simulink model "MotorPlant_23_lab2_discrete"  (R2019b)
settings: Solver=FixedStepAuto  StartTime=0.0  StopTime=2  FixedStep=0.001  RelTol=1e-3
settings Model: Creator=cmcaradi  LastModifiedBy=Laura

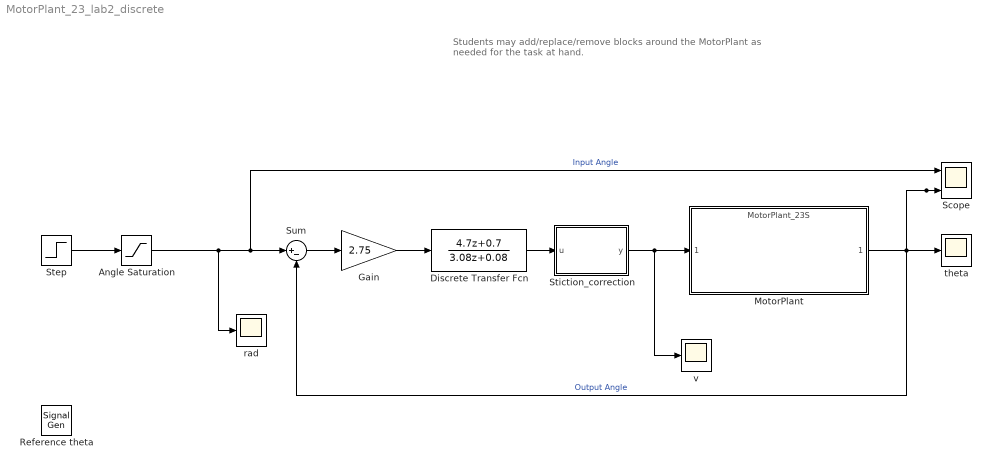
== system MotorPlant_23_lab2_discrete ==
  note: Students may add/replace/remove blocks around the
      | MotorPlant as needed for the task at hand.
  Angle Saturation : Saturate  UpperLimit=0.7  LowerLimit=-0.7
  Discrete Transfer Fcn : DiscreteTransferFcn  Numerator=[4.7 0.7]  Denominator=[3.08 0.08]  SampleTime=0.03
  Gain : Gain  Gain=2.75
  MotorPlant : ModelReference  ModelNameDialog=MotorPlant_23S  ModelReferenceVersion=1.41  CopyOfModelProtected=on
  Reference theta : SignalGenerator  WaveForm=square  Amplitude=45  Frequency=0.5
  Scope : Scope  NumInputPorts=2
  Step : Step  Before=-0.7  After=0.7  SampleTime=0
  Stiction_correction : MATLAB Function  TreatAsAtomicUnit=on
  Sum : Sum  Inputs=|+-
  rad : Scope
  theta : Scope
  v : Scope
  wires:
  MotorPlant/1 -> Scope/2, Sum/2, theta/1  "Output Angle"
  Angle Saturation/1 -> rad/1, Scope/1, Sum/1  "Input Angle"
  Stiction_correction/1(y) -> v/1, MotorPlant/1
  Discrete Transfer Fcn/1 -> Stiction_correction/1(u)
  Sum/1 -> Gain/1
  Gain/1 -> Discrete Transfer Fcn/1
  Step/1 -> Angle Saturation/1

== matlab function MotorPlant_23_lab2_discrete/Stiction_correction ==
  data: u input; y output
function y = fcn(u)

a = -0.48;
b = 0.50;

if u < b && u > 0
    y = u + b;
elseif u > a && u < 0
    y = u + a;
else
    y = u;

end
